simulink model "Subsystem"  (R2020b)
settings: Solver=VariableStepAuto  StartTime=0.0  StopTime=10.0  RelTol=1e-3
settings Model: Creator=Admin  LastModifiedBy=Admin
settings DataIOCC: SaveOutput=off  SaveTime=off

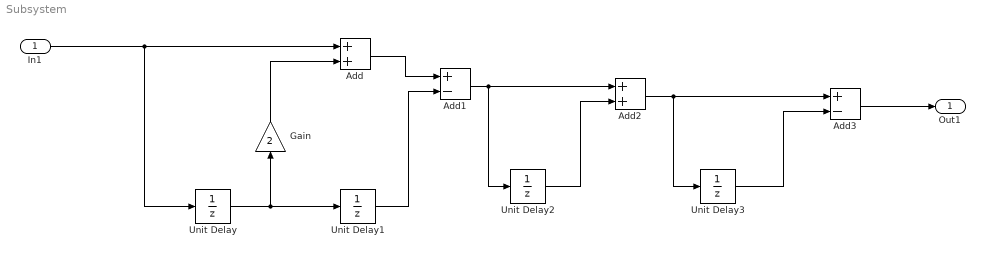
== system Subsystem ==
  In1 : Inport  OutDataTypeStr=double  PortDimensions=1  SampleTime=[0,1]
  Add : Sum
  Add1 : Sum  Inputs=+-
  Add2 : Sum
  Add3 : Sum  Inputs=+-
  Gain : Gain  Gain=2
  Unit Delay{,1..3} (4 alike) : UnitDelay  SampleTime=-1  HasFrameUpgradeWarning=on
  Out1 : Outport  OutDataTypeStr=double  PortDimensions=1  SampleTime=[0,1]
  wires:
  In1/1 -> Add/1, Unit Delay/1
  Unit Delay2/1 -> Add2/2
  Gain/1 -> Add/2
  Add2/1 -> Unit Delay3/1, Add3/1
  Add/1 -> Add1/1
  Add3/1 -> Out1/1
  Unit Delay3/1 -> Add3/2
  Unit Delay/1 -> Unit Delay1/1, Gain/1
  Unit Delay1/1 -> Add1/2
  Add1/1 -> Add2/1, Unit Delay2/1
